simulink model "Observer_7D"  (R2022a)
settings: Solver=VariableStepAuto  StartTime=0.0  StopTime=100  RelTol=1e-3
undefined symbols (not defined in the file): A, B, C, F, G, H, L
settings Model: Creator=thana  LastModifiedBy=hhaus

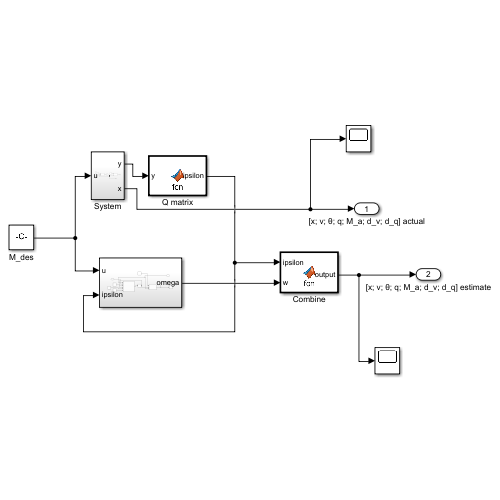
[thumbnail: Simulink's stored preview of the top-level diagram]
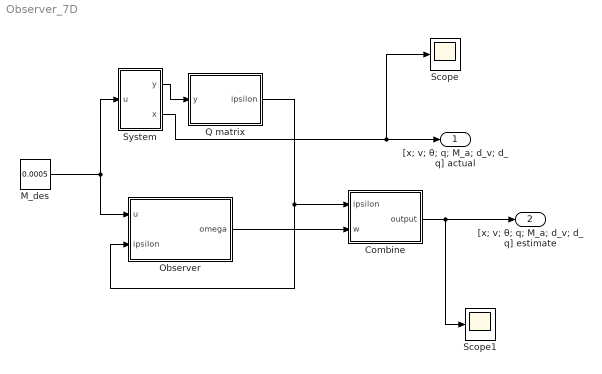
== system Observer_7D ==
  Combine : MATLAB Function  TreatAsAtomicUnit=on
  M_des : Constant  Value=0.0005
  Observer : Subsystem
  Q matrix : MATLAB Function  TreatAsAtomicUnit=on
  Scope : Scope
  Scope1 : Scope
  System : Subsystem
  "[x; v; θ; q; M_a; d_v; d_q] actual" : Outport
  "[x; v; θ; q; M_a; d_v; d_q] estimate" : Outport  Port=2
  wires:
  System/2(x) -> Scope/1, "[x; v; θ; q; M_a; d_v; d_q] actual"/1
  Q matrix/1(ipsilon) -> Combine/1(ipsilon), Observer/2(ipsilon)
  Combine/1(output) -> Scope1/1, "[x; v; θ; q; M_a; d_v; d_q] estimate"/1
  Observer/1(omega) -> Combine/2(w)
  M_des/1 -> Observer/1(u), System/1(u)
  System/1(y) -> Q matrix/1(y)

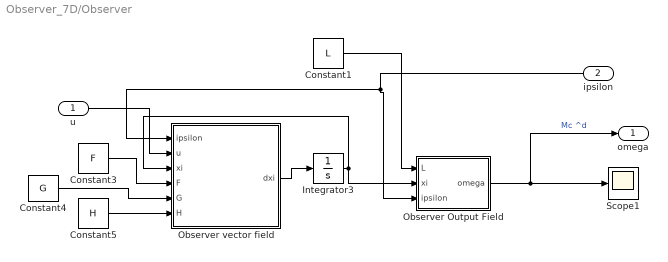
== system Observer_7D/Observer ==
  u : Inport
  ipsilon : Inport  Port=2
  Constant1 : Constant  Value=L
  Constant3 : Constant  Value=F
  Constant4 : Constant  Value=G
  Constant5 : Constant  Value=H
  Integrator3 : Integrator  InitialCondition=[0; 0; 0]
  Observer Output Field : MATLAB Function  TreatAsAtomicUnit=on
  Observer vector field : MATLAB Function  TreatAsAtomicUnit=on
  Scope1 : Scope
  omega : Outport
  wires:
  u/1 -> Observer vector field/2(u)
  Integrator3/1 -> Observer vector field/3(xi), Observer Output Field/2(xi)
  ipsilon/1 -> Observer Output Field/3(ipsilon), Observer vector field/1(ipsilon)
  Constant5/1 -> Observer vector field/6(H)
  Observer vector field/1(dxi) -> Integrator3/1
  Constant4/1 -> Observer vector field/5(G)
  Constant3/1 -> Observer vector field/4(F)
  Observer Output Field/1(omega) -> Scope1/1, omega/1  "Mc ^d"
  Constant1/1 -> Observer Output Field/1(L)

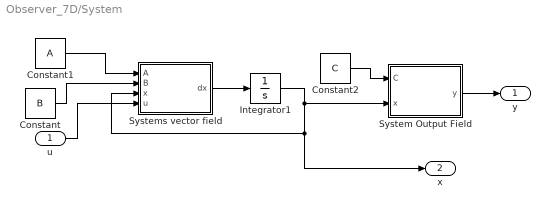
== system Observer_7D/System ==
  u : Inport
  Constant : Constant  Value=B
  Constant1 : Constant  Value=A
  Constant2 : Constant  Value=C
  Integrator1 : Integrator  InitialCondition=[0;0;0;0;0;0;0]
  System Output Field : MATLAB Function  TreatAsAtomicUnit=on
  Systems vector field : MATLAB Function  TreatAsAtomicUnit=on
  y : Outport
  x : Outport  Port=2
  wires:
  Systems vector field/1(dx) -> Integrator1/1
  Constant1/1 -> Systems vector field/1(A)
  Constant2/1 -> System Output Field/1(C)
  u/1 -> Systems vector field/4(u)
  Integrator1/1 -> x/1, Systems vector field/3(x), System Output Field/2(x)
  System Output Field/1(y) -> y/1
  Constant/1 -> Systems vector field/2(B)

== matlab function Observer_7D/Combine ==
  data: ipsilon input; output output; w input
function output = fcn(ipsilon, w)

output = [ipsilon;w];

== matlab function Observer_7D/Observer/Observer Output Field ==
  data: L input; xi input; omega output; ipsilon input
function omega = fcn(L, xi, ipsilon)

omega = xi + L*ipsilon;

== matlab function Observer_7D/Observer/Observer vector field ==
  data: ipsilon input; u input; dxi output; xi input; F input; G input; H input
function dxi = fcn(ipsilon,u, xi, F, G, H)

dxi = F*xi + H*ipsilon + G*u;

== matlab function Observer_7D/Q matrix ==
  data: y input; ipsilon output
function ipsilon = fcn(y)

ipsilon = y;

== matlab function Observer_7D/System/System Output Field ==
  data: C input; x input; y output
function y = fcn(C, x)

y = C*x;

== matlab function Observer_7D/System/Systems vector field ==
  data: A input; B input; x input; u input; dx output
function dx = fcn(A, B, x, u)

dx = (A*x) + (B*u);
